simulink model "gmStateSpaceHDL_pfc_desktop"  (R2024b)
settings: Solver=FixedStepDiscrete  StartTime=0.0  StopTime=.4  RelTol=1e-3
InitFcn:
  | fidelity_pfc_vals;
  | load('C:\Users\angro\Desktop\hil\pfc3ph\matlab\sim\sschdl\pfc_desktop\stateSpaceParameters.mat');
values from neighbouring files (symbols this model uses):
  fsw = 65    [fidelity_pfc_vals.m]
  Gs = 2e-2    (= 0.02)    [fidelity_pfc_vals.m]    (also in workspace.mat)
  s = 1    [fidelity_pfc_vals.m]    (also in workspace.mat)
  stateSpaceParameters_1 =     [workspace.mat]
  t_ss = tsw/35    (= 4.3956043956e-07)    [fidelity_pfc_vals.m]    (also in workspace.mat)
  tsw = 1/(fsw*1e3)    (= 1.53846153846e-05)    [fidelity_pfc_vals.m]    (also in workspace.mat)
undefined symbols (not defined in the file or in its folder): a, b, c, DiscIntNeverNeededParam
libraries: mcbcontrolslib x5, dspsrcs4 x3, simulink x2, slpidlib x2, hdlssclib x2, spsSVPWMGenerator2LevelLib x1, spsPLL3phLib x1, hdlsllib x1
CloseFcn:
  | clear stateSpaceParameters_1
settings Model: DataTypeOverride=Off  Creator=angro  LastModifiedBy=angro
settings OptimizationCC: BlockReduction=off  ConditionallyExecuteInputs=off  DefaultParameterBehavior=Inlined  InheritOutputTypeSmallerThanSingle=on
settings DebuggingCC: ArtificialAlgebraicLoopMsg=error  SingleTaskRateTransMsg=error
settings HardwareCC: ProdBitPerPointer=32  ProdBitPerSizeT=32  ProdBitPerPtrDiffT=32  ProdLargestAtomicFloat=None  ProdIntDivRoundTo=Undefined  ProdEndianess=Unspecified  ProdWordSize=32  ProdHWDeviceType=ASIC/FPGA->ASIC/FPGA  TargetBitPerPointer=64  TargetBitPerSizeT=64  TargetBitPerPtrDiffT=64  TargetLongLongMode=on  TargetIntDivRoundTo=Zero  TargetEndianess=LittleEndian  TargetWordSize=64  TargetHWDeviceType=Custom Processor->MATLAB Host Computer  ProdEqTarget=off

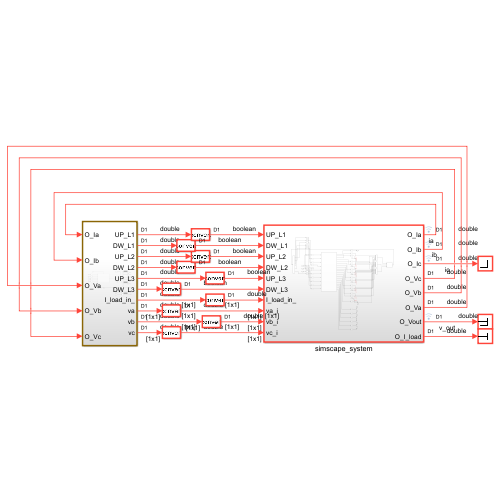
[thumbnail: Simulink's stored preview of the top-level diagram]
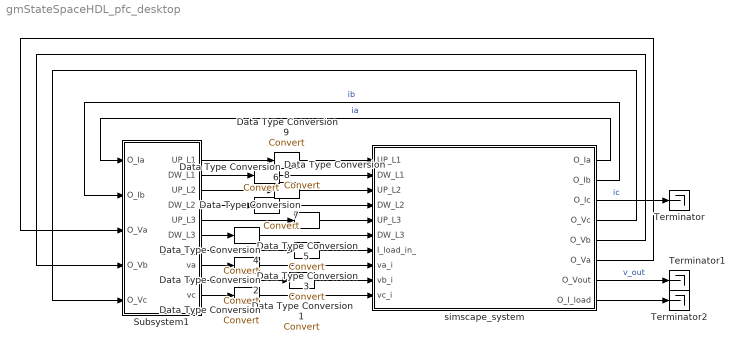
== system gmStateSpaceHDL_pfc_desktop ==
  Data Type Conversion{,1..9} (10 alike) : DataTypeConversion  SaturateOnIntegerOverflow=off  RndMeth=Floor
  Subsystem1 : Subsystem
  Terminator : Terminator
  Terminator1 : Terminator
  Terminator2 : Terminator
  simscape_system : Subsystem
  wires:
  simscape_system/1(O_Ia) -> Subsystem1/1(O_Ia)  "ia"
  simscape_system/2(O_Ib) -> Subsystem1/2(O_Ib)  "ib"
  simscape_system/3(O_Ic) -> Terminator/1  "ic"
  simscape_system/4(O_Vc) -> Subsystem1/5(O_Vc)
  simscape_system/5(O_Vb) -> Subsystem1/4(O_Vb)
  simscape_system/6(O_Va) -> Subsystem1/3(O_Va)
  Subsystem1/7(I_load_in_) -> Data Type Conversion3/1
  Subsystem1/1(UP_L1) -> Data Type Conversion9/1
  Subsystem1/2(DW_L1) -> Data Type Conversion8/1
  Subsystem1/3(UP_L2) -> Data Type Conversion7/1
  Subsystem1/4(DW_L2) -> Data Type Conversion6/1
  Subsystem1/5(UP_L3) -> Data Type Conversion5/1
  Subsystem1/6(DW_L3) -> Data Type Conversion4/1
  simscape_system/7(O_Vout) -> Terminator1/1  "v_out"
  Subsystem1/8(va) -> Data Type Conversion2/1
  Subsystem1/9(vb) -> Data Type Conversion1/1
  Subsystem1/10(vc) -> Data Type Conversion/1
  simscape_system/8(O_I_load) -> Terminator2/1
  Data Type Conversion/1 -> simscape_system/10(vc_i)
  Data Type Conversion1/1 -> simscape_system/9(vb_i)
  Data Type Conversion2/1 -> simscape_system/8(va_i)
  Data Type Conversion3/1 -> simscape_system/7(I_load_in_)
  Data Type Conversion4/1 -> simscape_system/6(DW_L3)
  Data Type Conversion5/1 -> simscape_system/5(UP_L3)
  Data Type Conversion6/1 -> simscape_system/4(DW_L2)
  Data Type Conversion7/1 -> simscape_system/3(UP_L2)
  Data Type Conversion8/1 -> simscape_system/2(DW_L1)
  Data Type Conversion9/1 -> simscape_system/1(UP_L1)

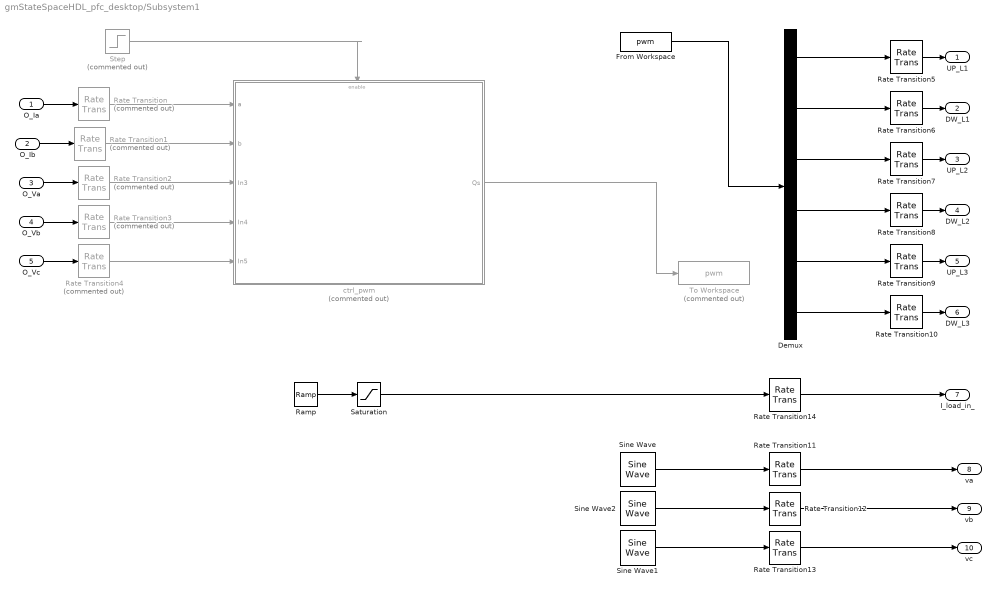
== system gmStateSpaceHDL_pfc_desktop/Subsystem1 ==
  O_Ia : Inport
  O_Ib : Inport  Port=2
  O_Va : Inport  Port=3
  O_Vb : Inport  Port=4
  O_Vc : Inport  Port=5
  Demux : Demux  Outputs=6
  From Workspace : FromWorkspace  VariableName=pwm  SampleTime=t_ss  Interpolate=off  ZeroCross=off  OutputAfterFinalValue=Holding final value
  Ramp : simulink/Sources/Ramp  slope=1/50  start=2/50  InitialOutput=0
  Rate Transition{,1..4} (5 alike) : RateTransition  Commented=on  OutPortSampleTime=t_ss
  Rate Transition{5..10,14} (7 alike) : RateTransition  OutPortSampleTime=t_ss
  Rate Transition11 : RateTransition
  Rate Transition12 : RateTransition
  Rate Transition13 : RateTransition
  Saturation : Saturate  UpperLimit=2
  Sine Wave : dspsrcs4/Sine Wave  Amplitude=325  Frequency=50  Phase=0  SampleMode=Discrete  OutComplex=Real  CompMethod=Table lookup  TableSize=Speed  SampleTime=tsw  SamplesPerFrame=1  ResetState=Restart at time zero  OutputFrames=off  dataType=double  wordLen=16  udDataType=sfix(16)  fracBitsMode=Best precision  numFracBits=15  OutDataTypeStr=double  LastOutDataTypeStr=double
  Sine Wave1 : dspsrcs4/Sine Wave  Amplitude=325  Frequency=50  Phase=2*pi/3  SampleMode=Discrete  OutComplex=Real  CompMethod=Table lookup  TableSize=Speed  SampleTime=tsw  SamplesPerFrame=1  ResetState=Restart at time zero  OutputFrames=off  dataType=double  wordLen=16  udDataType=sfix(16)  fracBitsMode=Best precision  numFracBits=15  OutDataTypeStr=double  LastOutDataTypeStr=double
  Sine Wave2 : dspsrcs4/Sine Wave  Amplitude=325  Frequency=50  Phase=-2*pi/3  SampleMode=Discrete  OutComplex=Real  CompMethod=Table lookup  TableSize=Speed  SampleTime=tsw  SamplesPerFrame=1  ResetState=Restart at time zero  OutputFrames=off  dataType=double  wordLen=16  udDataType=sfix(16)  fracBitsMode=Best precision  numFracBits=15  OutDataTypeStr=double  LastOutDataTypeStr=double
  Step : Step  Commented=on  Time=2/50  SampleTime=0
  To Workspace : ToWorkspace  Commented=on  VariableName=pwm  SaveFormat=Timeseries  SampleTime=-1
  ctrl_pwm : Subsystem  Commented=on
  UP_L1 : Outport
  DW_L1 : Outport  Port=2
  UP_L2 : Outport  Port=3
  DW_L2 : Outport  Port=4
  UP_L3 : Outport  Port=5
  DW_L3 : Outport  Port=6
  I_load_in_ : Outport  Port=7
  va : Outport  Port=8
  vb : Outport  Port=9
  vc : Outport  Port=10
  wires:
  Demux/5 -> Rate Transition9/1
  Demux/1 -> Rate Transition5/1
  Demux/6 -> Rate Transition10/1
  Demux/4 -> Rate Transition8/1
  Demux/3 -> Rate Transition7/1
  Demux/2 -> Rate Transition6/1
  O_Ia/1 -> Rate Transition/1
  O_Ib/1 -> Rate Transition1/1
  O_Va/1 -> Rate Transition2/1
  O_Vb/1 -> Rate Transition3/1
  O_Vc/1 -> Rate Transition4/1
  Rate Transition5/1 -> UP_L1/1
  Rate Transition6/1 -> DW_L1/1
  Rate Transition7/1 -> UP_L2/1
  Rate Transition8/1 -> DW_L2/1
  Rate Transition9/1 -> UP_L3/1
  Rate Transition10/1 -> DW_L3/1
  Saturation/1 -> Rate Transition14/1
  Sine Wave/1 -> Rate Transition11/1
  Sine Wave2/1 -> Rate Transition12/1
  Sine Wave1/1 -> Rate Transition13/1
  Rate Transition11/1 -> va/1
  Rate Transition12/1 -> vb/1
  Rate Transition13/1 -> vc/1
  ctrl_pwm/1(Qs) -> To Workspace/1
  Rate Transition/1 -> ctrl_pwm/1(a)
  Rate Transition1/1 -> ctrl_pwm/2(b)
  Rate Transition2/1 -> ctrl_pwm/3(In3)
  Rate Transition3/1 -> ctrl_pwm/4(In4)
  Rate Transition4/1 -> ctrl_pwm/5(In5)
  Step/1 -> ctrl_pwm/Enable
  Rate Transition14/1 -> I_load_in_/1
  Ramp/1 -> Saturation/1
  From Workspace/1 -> Demux/1

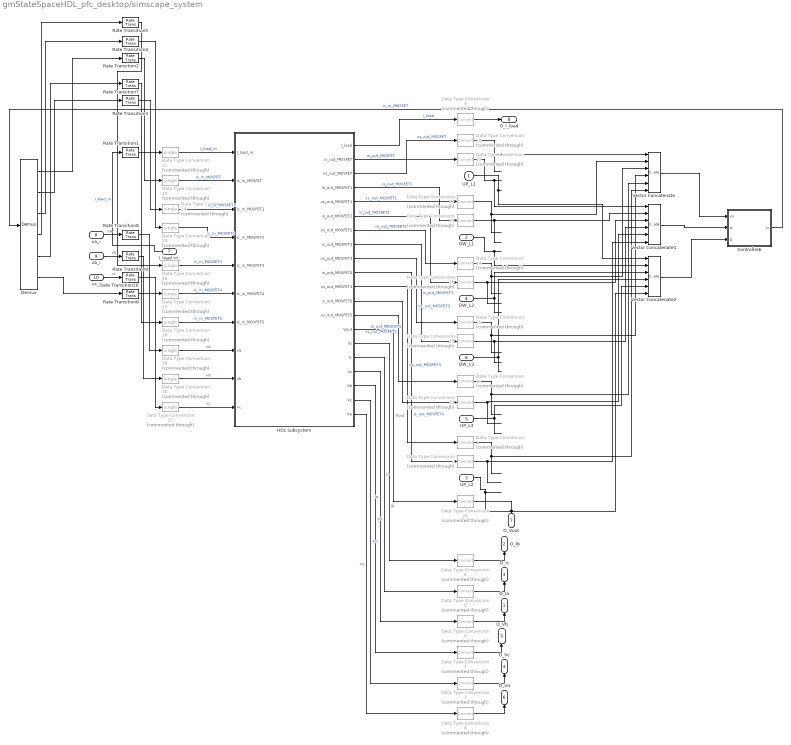
== system gmStateSpaceHDL_pfc_desktop/simscape_system ==
  UP_L1 : Inport
  DW_L1 : Inport  Port=2
  UP_L2 : Inport  Port=3
  DW_L2 : Inport  Port=4
  UP_L3 : Inport  Port=5
  DW_L3 : Inport  Port=6
  I_load_in_ : Inport  Port=7
  va_i : Inport  Port=8  LockScale=on
  vb_i : Inport  Port=9  LockScale=on
  vc_i : Inport  Port=10  LockScale=on
  Controller6 : Subsystem
  Data Type Conversion{1..20} (20 alike) : DataTypeConversion  Commented=through  RndMeth=Nearest  SaturateOnIntegerOverflow=off  LockScale=on
  Data Type Conversion{21..30} (10 alike) : DataTypeConversion  Commented=through  OutDataTypeStr=single  RndMeth=Nearest  SaturateOnIntegerOverflow=off
  Demux : Demux  Outputs=6
  HDL Subsystem : Subsystem
  Rate Transition{1..10} (10 alike) : RateTransition  OutPortSampleTime=4.395604395604395e-07
  Vector Concatenate : Concatenate  NumInputs=6
  Vector Concatenate1 : Concatenate  NumInputs=6
  Vector Concatenate2 : Concatenate  NumInputs=6
  O_Ia : Outport
  O_Ib : Outport  Port=2
  O_Ic : Outport  Port=3
  O_Vc : Outport  Port=4
  O_Vb : Outport  Port=5
  O_Va : Outport  Port=6
  O_Vout : Outport  Port=7
  O_I_load : Outport  Port=8
  wires:
  Data Type Conversion25/1 -> HDL Subsystem/4(ic_in_MOSFET2)  "ic_in_MOSFET2"
  Rate Transition3/1 -> Data Type Conversion24/1
  DW_L3/1 -> Vector Concatenate2/4
  va_i/1 -> Rate Transition8/1  "va"
  DW_L2/1 -> Vector Concatenate2/3
  Data Type Conversion12/1 -> Vector Concatenate1/1
  HDL Subsystem/2(is_out_MOSFET) -> Data Type Conversion12/1  "is_out_MOSFET"
  vc_i/1 -> Rate Transition10/1  "vc"
  I_load_in_/1 -> Rate Transition1/1  "I_load_in"
  UP_L2/1 -> Vector Concatenate2/6
  UP_L3/1 -> Vector Concatenate2/5
  vb_i/1 -> Rate Transition9/1  "vb"
  Rate Transition5/1 -> Data Type Conversion26/1
  Rate Transition4/1 -> Data Type Conversion25/1
  Data Type Conversion22/1 -> HDL Subsystem/10(vc)  "vc"
  Data Type Conversion2/1 -> Vector Concatenate1/6
  Data Type Conversion26/1 -> HDL Subsystem/5(ic_in_MOSFET3)  "ic_in_MOSFET3"
  Data Type Conversion18/1 -> Vector Concatenate1/4
  Rate Transition2/1 -> Data Type Conversion23/1
  Rate Transition7/1 -> Data Type Conversion28/1
  Data Type Conversion16/1 -> Vector Concatenate1/3
  HDL Subsystem/11(vs_out_MOSFET4) -> Data Type Conversion1/1  "vs_out_MOSFET4"
  Rate Transition1/1 -> Data Type Conversion21/1
  Rate Transition8/1 -> Data Type Conversion29/1
  Rate Transition9/1 -> Data Type Conversion30/1
  Rate Transition10/1 -> Data Type Conversion22/1
  Data Type Conversion8/1 -> O_Va/1
  Rate Transition6/1 -> Data Type Conversion27/1
  Data Type Conversion21/1 -> HDL Subsystem/1(I_load_in)  "I_load_in"
  Data Type Conversion20/1 -> O_Vout/1
  Data Type Conversion23/1 -> HDL Subsystem/2(ic_in_MOSFET)  "ic_in_MOSFET"
  HDL Subsystem/10(is_out_MOSFET4) -> Data Type Conversion2/1  "is_out_MOSFET4"
  Data Type Conversion24/1 -> HDL Subsystem/3(ic_in_MOSFET1)  "ic_in_MOSFET1"
  Data Type Conversion14/1 -> Vector Concatenate/3
  Data Type Conversion27/1 -> HDL Subsystem/6(ic_in_MOSFET4)  "ic_in_MOSFET4"
  Data Type Conversion28/1 -> HDL Subsystem/7(ic_in_MOSFET5)  "ic_in_MOSFET5"
  Data Type Conversion29/1 -> HDL Subsystem/8(va)  "va"
  HDL Subsystem/8(is_out_MOSFET3) -> Data Type Conversion18/1  "is_out_MOSFET3"
  Data Type Conversion30/1 -> HDL Subsystem/9(vb)  "vb"
  HDL Subsystem/1(I_load) -> Data Type Conversion9/1  "I_load"
  HDL Subsystem/3(vs_out_MOSFET) -> Data Type Conversion10/1  "vs_out_MOSFET"
  HDL Subsystem/4(is_out_MOSFET1) -> Data Type Conversion19/1  "is_out_MOSFET1"
  HDL Subsystem/5(vs_out_MOSFET1) -> Data Type Conversion17/1  "vs_out_MOSFET1"
  HDL Subsystem/6(is_out_MOSFET2) -> Data Type Conversion16/1  "is_out_MOSFET2"
  HDL Subsystem/7(vs_out_MOSFET2) -> Data Type Conversion14/1  "vs_out_MOSFET2"
  HDL Subsystem/9(vs_out_MOSFET3) -> Data Type Conversion15/1  "vs_out_MOSFET3"
  HDL Subsystem/12(is_out_MOSFET5) -> Data Type Conversion13/1  "is_out_MOSFET5"
  HDL Subsystem/13(vs_out_MOSFET5) -> Data Type Conversion11/1  "vs_out_MOSFET5"
  HDL Subsystem/14(Vout) -> Data Type Conversion20/1  "Vout"
  Data Type Conversion15/1 -> Vector Concatenate/4
  HDL Subsystem/15(Ib) -> Data Type Conversion6/1  "Ib"
  HDL Subsystem/16(Ic) -> Data Type Conversion5/1  "Ic"
  HDL Subsystem/17(Ia) -> Data Type Conversion4/1  "Ia"
  HDL Subsystem/18(Vb) -> Data Type Conversion7/1  "Vb"
  HDL Subsystem/19(Vc) -> Data Type Conversion3/1  "Vc"
  HDL Subsystem/20(Va) -> Data Type Conversion8/1  "Va"
  Data Type Conversion9/1 -> O_I_load/1
  Data Type Conversion13/1 -> Vector Concatenate1/5
  Data Type Conversion10/1 -> Vector Concatenate/1
  DW_L1/1 -> Vector Concatenate2/2
  UP_L1/1 -> Vector Concatenate2/1
  Data Type Conversion17/1 -> Vector Concatenate/2
  Data Type Conversion19/1 -> Vector Concatenate1/2
  Data Type Conversion11/1 -> Vector Concatenate/5
  Data Type Conversion1/1 -> Vector Concatenate/6
  Data Type Conversion6/1 -> O_Ib/1
  Data Type Conversion5/1 -> O_Ic/1
  Data Type Conversion4/1 -> O_Ia/1
  Data Type Conversion7/1 -> O_Vb/1
  Data Type Conversion3/1 -> O_Vc/1
  Vector Concatenate/1 -> Controller6/1(vs)
  Vector Concatenate1/1 -> Controller6/2(is)
  Vector Concatenate2/1 -> Controller6/3(G)
  Demux/1 -> Rate Transition2/1
  Demux/2 -> Rate Transition3/1
  Demux/3 -> Rate Transition4/1
  Demux/4 -> Rate Transition5/1
  Demux/5 -> Rate Transition7/1
  Demux/6 -> Rate Transition6/1
  Controller6/1(ic) -> Demux/1  "ic_in_MOSFET"

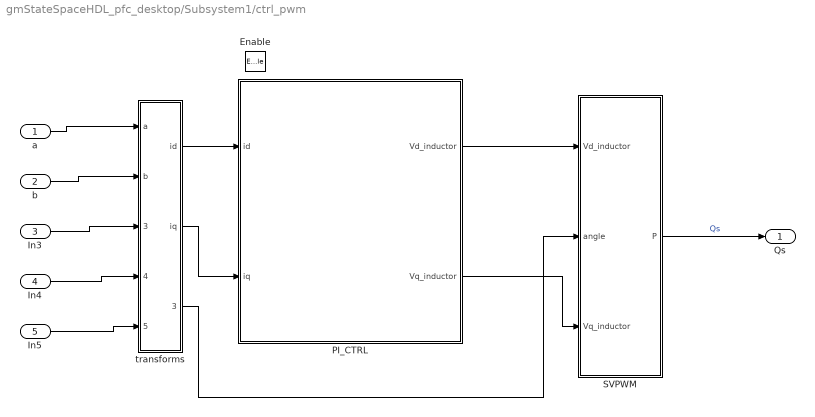
== system gmStateSpaceHDL_pfc_desktop/Subsystem1/ctrl_pwm ==
  a : Inport
  b : Inport  Port=2
  In3 : Inport  Port=3
  In4 : Inport  Port=4
  In5 : Inport  Port=5
  Enable : EnablePort
  PI_CTRL : Subsystem
  SVPWM : Subsystem
  transforms : Subsystem
  Qs : Outport
  wires:
  transforms/1(id) -> PI_CTRL/1(id)
  transforms/3(angle) -> SVPWM/2(angle)
  PI_CTRL/1(Vd_inductor) -> SVPWM/1(Vd_inductor)
  a/1 -> transforms/1(a)
  In5/1 -> transforms/5(In5)
  transforms/2(iq) -> PI_CTRL/2(iq)
  SVPWM/1(P) -> Qs/1  "Qs"
  PI_CTRL/2(Vq_inductor) -> SVPWM/3(Vq_inductor)
  b/1 -> transforms/2(b)
  In3/1 -> transforms/3(In3)
  In4/1 -> transforms/4(In4)

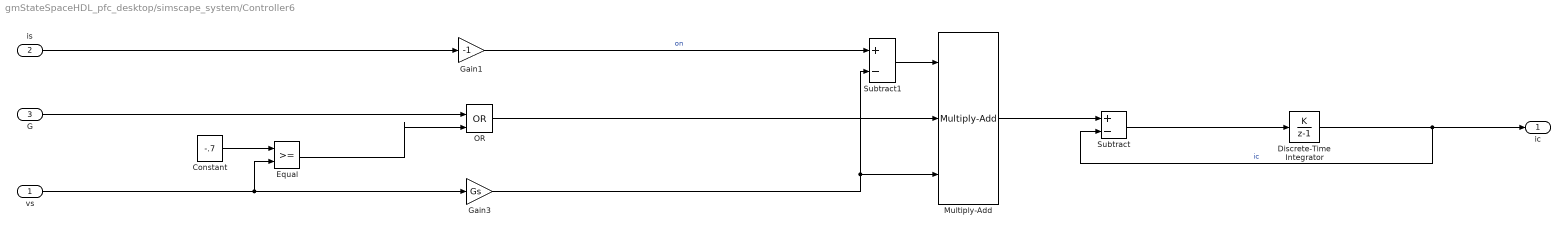
== system gmStateSpaceHDL_pfc_desktop/simscape_system/Controller6 ==
  vs : Inport
  is : Inport  Port=2
  G : Inport  Port=3
  Constant : Constant  Value=-.7  SampleTime=-1
  Discrete-Time Integrator : DiscreteIntegrator  IntegratorMethod=Accumulation: Forward Euler  gainval=1/s  SampleTime=-1  OutDataTypeStr=Inherit: Inherit via back propagation  ICPrevOutput=DiscIntNeverNeededParam  ICPrevScaledInput=DiscIntNeverNeededParam
  Equal : RelationalOperator  OutDataTypeStr=boolean  RndMeth=Simplest  InputSameDT=off
  Gain1 : Gain  Gain=-1  OutDataTypeStr=Inherit: Inherit via back propagation
  Gain3 : Gain  Gain=Gs  OutDataTypeStr=Inherit: Inherit via back propagation
  Multiply-Add : hdlsllib/HDL Operations/Multiply-Add  Function=c+(a.*b)  datatype=Inherit: Inherit via internal rule  DoSatur=off  FMA=off
  OR : Logic  Operator=OR  IconShape=distinctive  AllPortsSameDT=off  OutDataTypeStr=boolean
  Subtract : Sum  Inputs=+-
  Subtract1 : Sum  Inputs=+-
  ic : Outport
  wires:
  OR/1 -> Multiply-Add/2
  Subtract1/1 -> Multiply-Add/1
  Gain3/1 -> Multiply-Add/3, Subtract1/2
  Constant/1 -> Equal/1
  Equal/1 -> OR/2
  Subtract/1 -> Discrete-Time Integrator/1
  Discrete-Time Integrator/1 -> Subtract/2, ic/1  "ic"
  Gain1/1 -> Subtract1/1  "on"
  Multiply-Add/1 -> Subtract/1
  is/1 -> Gain1/1
  G/1 -> OR/1
  vs/1 -> Gain3/1, Equal/2

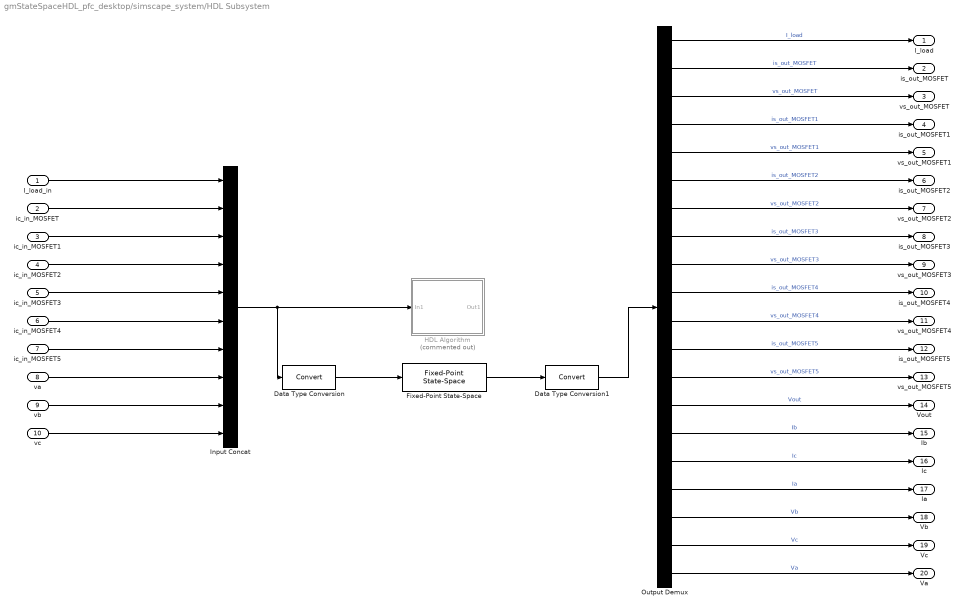
== system gmStateSpaceHDL_pfc_desktop/simscape_system/HDL Subsystem ==
  I_load_in : Inport
  ic_in_MOSFET : Inport  Port=2
  ic_in_MOSFET1 : Inport  Port=3
  ic_in_MOSFET2 : Inport  Port=4
  ic_in_MOSFET3 : Inport  Port=5
  ic_in_MOSFET4 : Inport  Port=6
  ic_in_MOSFET5 : Inport  Port=7
  va : Inport  Port=8
  vb : Inport  Port=9
  vc : Inport  Port=10
  Data Type Conversion : DataTypeConversion  SaturateOnIntegerOverflow=off  RndMeth=Floor
  Data Type Conversion1 : DataTypeConversion  SaturateOnIntegerOverflow=off  RndMeth=Floor
  Fixed-Point State-Space : simulink/Additional Math & Discrete/Additional Discrete/Fixed-Point State-Space  A=stateSpaceParameters_1.Ad  B=stateSpaceParameters_1.Bd  C=stateSpaceParameters_1.Cd  D=stateSpaceParameters_1.Dd  InitialCondition=stateSpaceParameters_1.X0  InternalDataType=fixdt('single')  StateEqScaling=2^0  OutputEqScaling=2^0  DoSatur=off
  HDL Algorithm : Subsystem  Commented=on
  Input Concat : Concatenate  NumInputs=10
  Output Demux : Demux  Outputs=20
  I_load : Outport
  is_out_MOSFET : Outport  Port=2
  vs_out_MOSFET : Outport  Port=3
  is_out_MOSFET1 : Outport  Port=4
  vs_out_MOSFET1 : Outport  Port=5
  is_out_MOSFET2 : Outport  Port=6
  vs_out_MOSFET2 : Outport  Port=7
  is_out_MOSFET3 : Outport  Port=8
  vs_out_MOSFET3 : Outport  Port=9
  is_out_MOSFET4 : Outport  Port=10
  vs_out_MOSFET4 : Outport  Port=11
  is_out_MOSFET5 : Outport  Port=12
  vs_out_MOSFET5 : Outport  Port=13
  Vout : Outport  Port=14
  Ib : Outport  Port=15
  Ic : Outport  Port=16
  Ia : Outport  Port=17
  Vb : Outport  Port=18
  Vc : Outport  Port=19
  Va : Outport  Port=20
  wires:
  Output Demux/7 -> vs_out_MOSFET2/1  "vs_out_MOSFET2"
  Output Demux/2 -> is_out_MOSFET/1  "is_out_MOSFET"
  Output Demux/3 -> vs_out_MOSFET/1  "vs_out_MOSFET"
  Output Demux/4 -> is_out_MOSFET1/1  "is_out_MOSFET1"
  ic_in_MOSFET/1 -> Input Concat/2
  Input Concat/1 -> Data Type Conversion/1, HDL Algorithm/1(In1)
  Output Demux/17 -> Ia/1  "Ia"
  Output Demux/1 -> I_load/1  "I_load"
  vc/1 -> Input Concat/10
  Output Demux/6 -> is_out_MOSFET2/1  "is_out_MOSFET2"
  Output Demux/8 -> is_out_MOSFET3/1  "is_out_MOSFET3"
  Output Demux/15 -> Ib/1  "Ib"
  Output Demux/13 -> vs_out_MOSFET5/1  "vs_out_MOSFET5"
  Output Demux/5 -> vs_out_MOSFET1/1  "vs_out_MOSFET1"
  Output Demux/12 -> is_out_MOSFET5/1  "is_out_MOSFET5"
  Output Demux/10 -> is_out_MOSFET4/1  "is_out_MOSFET4"
  Output Demux/9 -> vs_out_MOSFET3/1  "vs_out_MOSFET3"
  Output Demux/11 -> vs_out_MOSFET4/1  "vs_out_MOSFET4"
  Output Demux/14 -> Vout/1  "Vout"
  Output Demux/16 -> Ic/1  "Ic"
  Output Demux/19 -> Vc/1  "Vc"
  Output Demux/18 -> Vb/1  "Vb"
  Output Demux/20 -> Va/1  "Va"
  vb/1 -> Input Concat/9
  ic_in_MOSFET1/1 -> Input Concat/3
  I_load_in/1 -> Input Concat/1
  ic_in_MOSFET3/1 -> Input Concat/5
  ic_in_MOSFET2/1 -> Input Concat/4
  ic_in_MOSFET5/1 -> Input Concat/7
  va/1 -> Input Concat/8
  ic_in_MOSFET4/1 -> Input Concat/6
  Data Type Conversion/1 -> Fixed-Point State-Space/1
  Fixed-Point State-Space/1 -> Data Type Conversion1/1
  Data Type Conversion1/1 -> Output Demux/1

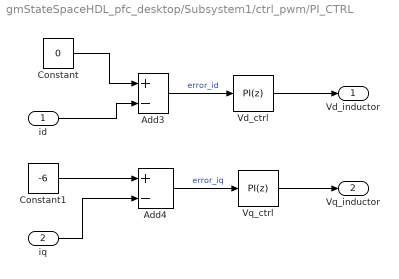
== system gmStateSpaceHDL_pfc_desktop/Subsystem1/ctrl_pwm/PI_CTRL ==
  id : Inport
  iq : Inport  Port=2
  Add3 : Sum  Inputs=+-
  Add4 : Sum  Inputs=+-
  Constant : Constant  Value=0  SampleTime=t_ss
  Constant1 : Constant  Value=-6  SampleTime=t_ss
  Vd_ctrl : slpidlib/PID Controller  Controller=PI  Form=Parallel  TimeDomain=Discrete-time  UseExternalTs=off  SampleTime=t_ss  IntegratorMethod=Backward Euler  FilterMethod=Forward Euler  ControllerParametersSource=internal  P=-1.8  I=-.15  UseKiTs=off  D=0  UseExternalDerivativeSource=off  N=100  UseFilter=on  TunerSelectOption=Transfer Function Based (PID Tuner App)  InitialConditionSource=internal  InitialConditionForIntegrator=0  InitialConditionForFilter=0  DifferentiatorICPrevScaledInput=0  ExternalReset=none  TrackingMode=off  Kt=1  LimitOutput=off  SatLimitsSource=internal  UpperSaturationLimit=5e2  LowerSaturationLimit=-5e2  LinearizeAsGain=on  AntiWindupMode=clamping  Kb=1  LimitIntegrator=off  UpperIntegratorSaturationLimit=inf  LowerIntegratorSaturationLimit=-inf  POutMin=[]  POutMax=[]  IOutMin=[]  IOutMax=[]  DOutMin=[]  DOutMax=[]  NOutMin=[]  NOutMax=[]  SumOutMin=[]  SumOutMax=[]  SaturationOutMin=[]  SaturationOutMax=[]  PParamMin=[]  PParamMax=[]  IParamMin=[]  IParamMax=[]  DParamMin=[]  DParamMax=[]  NParamMin=[]  NParamMax=[]  KbParamMin=[]  KbParamMax=[]  KtParamMin=[]  KtParamMax=[]  KbOutMin=[]  KbOutMax=[]  KtOutMin=[]  KtOutMax=[]  IntegratorOutMin=[]  IntegratorOutMax=[]  FilterOutMin=[]  FilterOutMax=[]  SumI1OutMin=[]  SumI1OutMax=[]  SumI2OutMin=[]  SumI2OutMax=[]  SumI3OutMin=[]  SumI3OutMax=[]  SumI4OutMin=[]  SumI4OutMax=[]  SumDOutMin=[]  SumDOutMax=[]  DifferentiatorOutMin=[]  DifferentiatorOutMax=[]  FilterDiffOutCoefMin=[]  FilterDiffOutCoefMax=[]  ReciprocalOutMin=[]  ReciprocalOutMax=[]  SumDenOutMin=[]  SumDenOutMax=[]  SumNumOutMin=[]  SumNumOutMax=[]  DivideOutMin=[]  DivideOutMax=[]  UdiffTsProdOutMin=[]  UdiffTsProdOutMax=[]  NTsProdOutMin=[]  NTsProdOutMax=[]  UintegralTsProdOutMin=[]  UintegralTsProdOutMax=[]  UngainTsProdOutMin=[]  UngainTsProdOutMax=[]  ClampingZeroOutDataTypeStr=Inherit: Inherit via back propagation  ClampingZeroOutMin=[]  ClampingZeroOutMax=[]  FilterDenConstantOutDataTypeStr=Inherit: Inherit via back propagation  FilterDenConstantOutMin=[]  FilterDenConstantOutMax=[]  PCopyOutDataTypeStr=Inherit: Inherit via back propagation  PCopyOutMin=[]  PCopyOutMax=[]  NCopyOutDataTypeStr=Inherit: Inherit via back propagation  NCopyOutMin=[]  NCopyOutMax=[]  IntegratorContinuousStateAttributes=''  IntegratorStateMustResolveToSignalObject=off  IntegratorRTWStateStorageClass=Auto  FilterContinuousStateAttributes=''  FilterStateMustResolveToSignalObject=off  FilterRTWStateStorageClass=Auto  ParallelPVariant=InternalParameters  IdealPVariant=Disabled  IVariant=InternalParameters  DVariant=Disabled  IntegratorVariant=Discrete  SatVariant=Disabled  AWVariant=Passthrough  PCopyVariant=Disabled  TRVariant=Disabled  FdbkBlocksVariant=Forward  IdealPFdbkVariant=Disabled  SatFdbkVariant=Disabled  DerivativeFilterVariant=Disabled  NVariant=Disabled  NCopyVariant=Disabled_SignalSpec  FilterICVariant=Disabled  IntegratorICVariant=InternalICs  ExternalResetVariant=Disabled  TRSumVariant=Passthrough  SumFdbkVariant=Disabled  SumVariant=Sum_PI  TsampFilterVariant=InternalTs  TsampNgainVariant=Passthrough  TsampIntegralVariant=Disabled_SignalSpec  ExternalSaturationOutDataTypeStr=Inherit: Same as second input  DerivativeSourceVariant=Disabled  PreIntVariant=InternalPreInt
  Vq_ctrl : slpidlib/PID Controller  Controller=PI  Form=Parallel  TimeDomain=Discrete-time  UseExternalTs=off  SampleTime=t_ss  IntegratorMethod=Backward Euler  FilterMethod=Forward Euler  ControllerParametersSource=internal  P=-2  I=-.2  UseKiTs=off  D=0  UseExternalDerivativeSource=off  N=100  UseFilter=on  TunerSelectOption=Transfer Function Based (PID Tuner App)  InitialConditionSource=internal  InitialConditionForIntegrator=0  InitialConditionForFilter=0  DifferentiatorICPrevScaledInput=0  ExternalReset=none  TrackingMode=off  Kt=1  LimitOutput=off  SatLimitsSource=internal  UpperSaturationLimit=5e2  LowerSaturationLimit=-5e2  LinearizeAsGain=on  AntiWindupMode=clamping  Kb=1  LimitIntegrator=off  UpperIntegratorSaturationLimit=inf  LowerIntegratorSaturationLimit=-inf  POutMin=[]  POutMax=[]  IOutMin=[]  IOutMax=[]  DOutMin=[]  DOutMax=[]  NOutMin=[]  NOutMax=[]  SumOutMin=[]  SumOutMax=[]  SaturationOutMin=[]  SaturationOutMax=[]  PParamMin=[]  PParamMax=[]  IParamMin=[]  IParamMax=[]  DParamMin=[]  DParamMax=[]  NParamMin=[]  NParamMax=[]  KbParamMin=[]  KbParamMax=[]  KtParamMin=[]  KtParamMax=[]  KbOutMin=[]  KbOutMax=[]  KtOutMin=[]  KtOutMax=[]  IntegratorOutMin=[]  IntegratorOutMax=[]  FilterOutMin=[]  FilterOutMax=[]  SumI1OutMin=[]  SumI1OutMax=[]  SumI2OutMin=[]  SumI2OutMax=[]  SumI3OutMin=[]  SumI3OutMax=[]  SumI4OutMin=[]  SumI4OutMax=[]  SumDOutMin=[]  SumDOutMax=[]  DifferentiatorOutMin=[]  DifferentiatorOutMax=[]  FilterDiffOutCoefMin=[]  FilterDiffOutCoefMax=[]  ReciprocalOutMin=[]  ReciprocalOutMax=[]  SumDenOutMin=[]  SumDenOutMax=[]  SumNumOutMin=[]  SumNumOutMax=[]  DivideOutMin=[]  DivideOutMax=[]  UdiffTsProdOutMin=[]  UdiffTsProdOutMax=[]  NTsProdOutMin=[]  NTsProdOutMax=[]  UintegralTsProdOutMin=[]  UintegralTsProdOutMax=[]  UngainTsProdOutMin=[]  UngainTsProdOutMax=[]  ClampingZeroOutDataTypeStr=Inherit: Inherit via back propagation  ClampingZeroOutMin=[]  ClampingZeroOutMax=[]  FilterDenConstantOutDataTypeStr=Inherit: Inherit via back propagation  FilterDenConstantOutMin=[]  FilterDenConstantOutMax=[]  PCopyOutDataTypeStr=Inherit: Inherit via back propagation  PCopyOutMin=[]  PCopyOutMax=[]  NCopyOutDataTypeStr=Inherit: Inherit via back propagation  NCopyOutMin=[]  NCopyOutMax=[]  IntegratorContinuousStateAttributes=''  IntegratorStateMustResolveToSignalObject=off  IntegratorRTWStateStorageClass=Auto  FilterContinuousStateAttributes=''  FilterStateMustResolveToSignalObject=off  FilterRTWStateStorageClass=Auto  ParallelPVariant=InternalParameters  IdealPVariant=Disabled  IVariant=InternalParameters  DVariant=Disabled  IntegratorVariant=Discrete  SatVariant=Disabled  AWVariant=Passthrough  PCopyVariant=Disabled  TRVariant=Disabled  FdbkBlocksVariant=Forward  IdealPFdbkVariant=Disabled  SatFdbkVariant=Disabled  DerivativeFilterVariant=Disabled  NVariant=Disabled  NCopyVariant=Disabled_SignalSpec  FilterICVariant=Disabled  IntegratorICVariant=InternalICs  ExternalResetVariant=Disabled  TRSumVariant=Passthrough  SumFdbkVariant=Disabled  SumVariant=Sum_PI  TsampFilterVariant=InternalTs  TsampNgainVariant=Passthrough  TsampIntegralVariant=Disabled_SignalSpec  ExternalSaturationOutDataTypeStr=Inherit: Same as second input  DerivativeSourceVariant=Disabled  PreIntVariant=InternalPreInt
  Vd_inductor : Outport
  Vq_inductor : Outport  Port=2
  wires:
  Add3/1 -> Vd_ctrl/1  "error_id"
  id/1 -> Add3/2
  Constant/1 -> Add3/1
  iq/1 -> Add4/2
  Add4/1 -> Vq_ctrl/1  "error_iq"
  Vd_ctrl/1 -> Vd_inductor/1
  Vq_ctrl/1 -> Vq_inductor/1
  Constant1/1 -> Add4/1

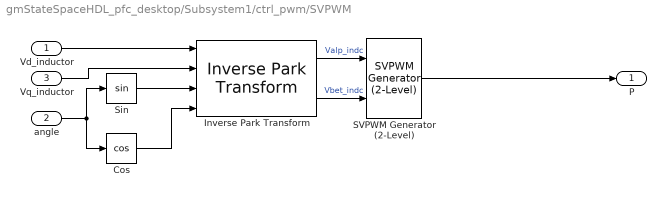
== system gmStateSpaceHDL_pfc_desktop/Subsystem1/ctrl_pwm/SVPWM ==
  Vd_inductor : Inport
  angle : Inport  Port=2
  Vq_inductor : Inport  Port=3
  Cos : Trigonometry  Operator=cos
  Inverse Park Transform : mcbcontrolslib/Inverse Park Transform  PhaseInput=Two inputs  AxisAlignment=D-axis  ThetaInput=Sine and Cosine electrical position  AngleInput=Per-unit  N_points=1024
  SVPWM Generator (2-Level) : spsSVPWMGenerator2LevelLib/SVPWM Generator (2-Level)  InputType=alpha-beta components  SwitchingPattern=Pattern #1  Fc=fsw*1e3  ParUref=[0.8 -30 50]  Ts=t_ss
  Sin : Trigonometry
  P : Outport
  wires:
  Vd_inductor/1 -> Inverse Park Transform/1
  Vq_inductor/1 -> Inverse Park Transform/2
  Inverse Park Transform/2 -> SVPWM Generator (2-Level)/2  "Vbet_indc"
  Sin/1 -> Inverse Park Transform/3
  Cos/1 -> Inverse Park Transform/4
  Inverse Park Transform/1 -> SVPWM Generator (2-Level)/1  "Valp_indc"
  angle/1 -> Cos/1, Sin/1
  SVPWM Generator (2-Level)/1 -> P/1

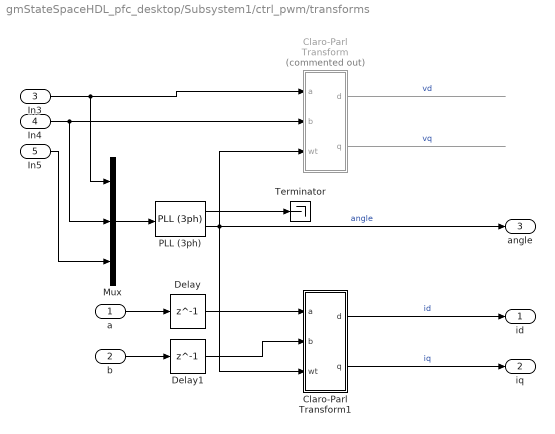
== system gmStateSpaceHDL_pfc_desktop/Subsystem1/ctrl_pwm/transforms ==
  a : Inport
  b : Inport  Port=2
  In3 : Inport  Port=3
  In4 : Inport  Port=4
  In5 : Inport  Port=5
  Claro-Parl Transform : Subsystem  Commented=on
  Claro-Parl Transform1 : Subsystem
  Delay : Delay  DelayLength=1
  Delay1 : Delay  DelayLength=1
  Mux : Mux  Inputs=3
  PLL (3ph) : spsPLL3phLib/PLL (3ph)  Fmin=50  Par_Init=[0, 50]  ParK=[180,3200,1]  TcD=1e-4  MaxRateChangeFreq=12  FilterCutOffFreq=25  Ts=t_ss  AGC=on
  Terminator : Terminator
  id : Outport
  iq : Outport  Port=2
  angle : Outport  Port=3
  wires:
  Mux/1 -> PLL (3ph)/1
  PLL (3ph)/2 -> angle/1, Claro-Parl Transform1/3(wt), Claro-Parl Transform/3(wt)  "angle"
  PLL (3ph)/1 -> Terminator/1
  In3/1 -> Mux/1, Claro-Parl Transform/1(a)
  In5/1 -> Mux/3
  b/1 -> Delay1/1
  In4/1 -> Claro-Parl Transform/2(b), Mux/2
  a/1 -> Delay/1
  Delay/1 -> Claro-Parl Transform1/1(a)
  Delay1/1 -> Claro-Parl Transform1/2(b)
  Claro-Parl Transform/1(d) -> ?  "vd"
  Claro-Parl Transform/2(q) -> ?  "vq"
  Claro-Parl Transform1/1(d) -> id/1  "id"
  Claro-Parl Transform1/2(q) -> iq/1  "iq"

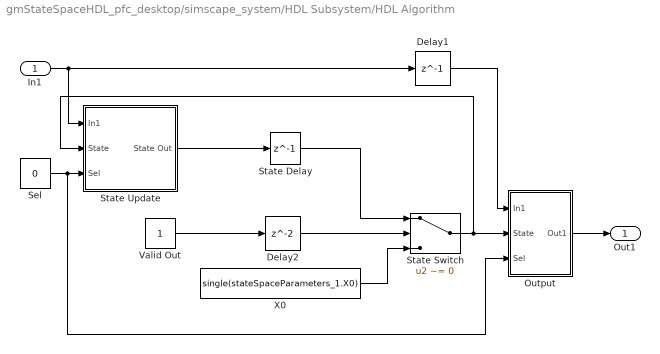
== system gmStateSpaceHDL_pfc_desktop/simscape_system/HDL Subsystem/HDL Algorithm ==
  In1 : Inport
  Delay1 : Delay  DelayLength=1
  Delay2 : Delay
  Output : Subsystem
  Sel : Constant  Value=0  OutDataTypeStr=uint32  SampleTime=-1
  State Delay : Delay  DelayLength=1  InitialCondition=single(stateSpaceParameters_1.X0)
  State Switch : Switch  Criteria=u2 ~= 0  SaturateOnIntegerOverflow=off  InputSameDT=off
  State Update : Subsystem
  Valid Out : Constant  OutDataTypeStr=boolean  SampleTime=4.395604395604395e-07
  X0 : Constant  Value=single(stateSpaceParameters_1.X0)  SampleTime=4.395604395604395e-07
  Out1 : Outport  VectorParamsAs1DForOutWhenUnconnected=off
  wires:
  Delay1/1 -> Output/1(In1)
  In1/1 -> Delay1/1, State Update/1(In1)
  Sel/1 -> Output/3(Sel), State Update/3(Sel)
  State Update/1(State Out) -> State Delay/1
  Valid Out/1 -> Delay2/1
  State Delay/1 -> State Switch/1
  Delay2/1 -> State Switch/2
  X0/1 -> State Switch/3
  State Switch/1 -> State Update/2(State), Output/2(State)
  Output/1(Out1) -> Out1/1

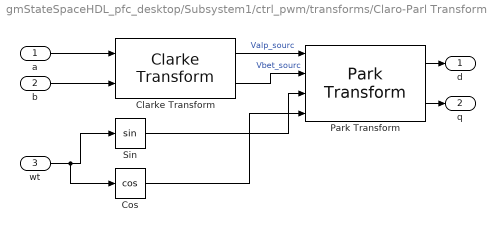
== system gmStateSpaceHDL_pfc_desktop/Subsystem1/ctrl_pwm/transforms/Claro-Parl Transform ==
  a : Inport
  b : Inport  Port=2
  wt : Inport  Port=3
  Clarke Transform : mcbcontrolslib/Clarke Transform  VariantControl=Variant2  PhaseInput=Two inputs  EnPowerInv=off
  Cos : Trigonometry  Operator=cos
  Park Transform : mcbcontrolslib/Park Transform  PhaseInput=Two inputs  AxisAlignment=D-axis  ThetaInput=Sine and Cosine electrical position  AngleInput=Per-unit  N_points=1024
  Sin : Trigonometry
  d : Outport
  q : Outport  Port=2
  wires:
  Clarke Transform/2 -> Park Transform/2  "Vbet_sourc"
  b/1 -> Clarke Transform/2
  Park Transform/2 -> q/1
  Park Transform/1 -> d/1
  Clarke Transform/1 -> Park Transform/1  "Valp_sourc"
  wt/1 -> Cos/1, Sin/1
  a/1 -> Clarke Transform/1
  Sin/1 -> Park Transform/3
  Cos/1 -> Park Transform/4

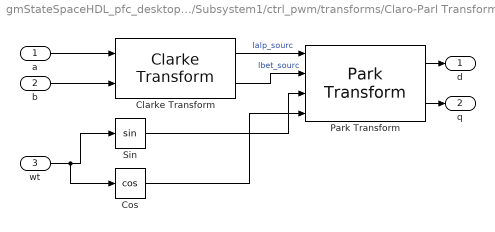
== system gmStateSpaceHDL_pfc_desktop/Subsystem1/ctrl_pwm/transforms/Claro-Parl Transform1 ==
  a : Inport
  b : Inport  Port=2
  wt : Inport  Port=3
  Clarke Transform : mcbcontrolslib/Clarke Transform  VariantControl=Variant2  PhaseInput=Two inputs  EnPowerInv=off
  Cos : Trigonometry  Operator=cos
  Park Transform : mcbcontrolslib/Park Transform  PhaseInput=Two inputs  AxisAlignment=D-axis  ThetaInput=Sine and Cosine electrical position  AngleInput=Per-unit  N_points=1024
  Sin : Trigonometry
  d : Outport
  q : Outport  Port=2
  wires:
  Clarke Transform/2 -> Park Transform/2  "Ibet_sourc"
  b/1 -> Clarke Transform/2
  Park Transform/2 -> q/1
  Park Transform/1 -> d/1
  Clarke Transform/1 -> Park Transform/1  "Ialp_sourc"
  wt/1 -> Cos/1, Sin/1
  a/1 -> Clarke Transform/1
  Sin/1 -> Park Transform/3
  Cos/1 -> Park Transform/4

== system gmStateSpaceHDL_pfc_desktop/simscape_system/HDL Subsystem/HDL Algorithm/Output ==
  In1 : Inport
  State : Inport  Port=2
  Sel : Inport  Port=3  LockScale=on
  Bias : Terminator
  Mux : Mux  Inputs=2
  Output Update : hdlssclib/NFPSparseConstMultiply  MatrixSource=Dialog  constMatrix=single([stateSpaceParameters_1.Cd stateSpaceParameters_1.Dd])  MatrixType=single  MatrixSize=[1 1]  ColumnIndices=[1]  RowIndices=[1]  PropDataType=single  defWL=48
  Out1 : Outport  VectorParamsAs1DForOutWhenUnconnected=off
  wires:
  State/1 -> Mux/1
  Mux/1 -> Output Update/1
  In1/1 -> Mux/2
  Sel/1 -> Bias/1, Output Update/2
  Output Update/1 -> Out1/1

== system gmStateSpaceHDL_pfc_desktop/simscape_system/HDL Subsystem/HDL Algorithm/State Update ==
  In1 : Inport
  State : Inport  Port=2
  Sel : Inport  Port=3  LockScale=on
  Bias : Terminator
  Mux : Mux  Inputs=2
  State Update : hdlssclib/NFPSparseConstMultiply  MatrixSource=Dialog  constMatrix=single([stateSpaceParameters_1.Ad stateSpaceParameters_1.Bd])  MatrixType=single  MatrixSize=[1 1]  ColumnIndices=[1]  RowIndices=[1]  PropDataType=single  defWL=48
  State Out : Outport  OutDataTypeStr=single  VectorParamsAs1DForOutWhenUnconnected=off
  wires:
  State/1 -> Mux/1
  In1/1 -> Mux/2
  Mux/1 -> State Update/1
  Sel/1 -> Bias/1, State Update/2
  State Update/1 -> State Out/1
